simulink library "libControlTrimInputs"  (R2020b)
settings: Solver=VariableStepAuto  StartTime=0.0  StopTime=10.0  RelTol=1e-3
settings Model: Creator=caatay  LastModifiedBy=caatay

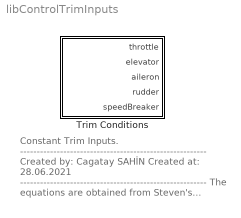
== system libControlTrimInputs ==
  note: Constant Trim Inputs.
      | --------------------------------------------------------
      | Created by: Cagatay SAHİN
      | Created at: 28.06.2021
      | --------------------------------------------------------
      | The equations are obtained from
      | Steven's textbook.
      | The reference book can be found in
      | "references folder".
      | --------------------------------------------------------
      | for question:
      | cagataysahin44@gmail.com
  Trim Conditions : Subsystem  mask(Flight Control System Model - Trim Input Library){throttle=outputs.trim.controls.throttle, elevator=outputs.trim.controls.elevator, aileron=outputs.trim.controls.aileron, rudder=outputs.trim.controls.rudder, sb=outputs.trim.controls.sb}
      mask prompts: throttle "Trimmed throttle value"; elevator "Trimmed elevator value"; aileron "Trimmed aileron value"; rudder "Trimmed rudder value"; sb "Trimmed sb value"
      mask help: Initialize trim input values for aircraft's steady-state flight
      mask Help:
      | This block is used for flight at steady-state trim inpıt.
      | --------------------------------------------------------------------------------------------------------------------------------------------------
      | Output of the function:
      | 	throttle: Trimmed throttle value.
      | 	elevator: Trimmed elevator value.
      | 	aileron: Trimmed aileron value.
      | 	rudder: Trimmed rudder value.
      | 	speedBreaker: Trimmed speedBreaker value.
      | --------------------------------------------------------------------------------------------------------------------------------------------------
      | All equations can be found in Steven's text book. Reference can be found in "literature" subfolder.
      | for question: "cagataysahin44@gmail.com"
      mask Display:
      | port_label('output',1,'\delta_{t}','texmode','on');
      | port_label('output',2,'\delta_{ele}','texmode','on');
      | port_label('output',3,'\delta_{ail}','texmode','on');
      | port_label('output',4,'\delta_{rud}','texmode','on');
      | port_label('output',5,'\delta_{sb}','texmode','on');

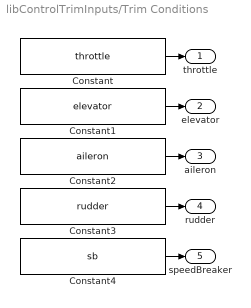
== system libControlTrimInputs/Trim Conditions ==
  Constant : Constant  Value=throttle
  Constant1 : Constant  Value=elevator
  Constant2 : Constant  Value=aileron
  Constant3 : Constant  Value=rudder
  Constant4 : Constant  Value=sb
  throttle : Outport  VectorParamsAs1DForOutWhenUnconnected=off
  elevator : Outport  Port=2  VectorParamsAs1DForOutWhenUnconnected=off
  aileron : Outport  Port=3  VectorParamsAs1DForOutWhenUnconnected=off
  rudder : Outport  Port=4  VectorParamsAs1DForOutWhenUnconnected=off
  speedBreaker : Outport  Port=5  VectorParamsAs1DForOutWhenUnconnected=off
  wires:
  Constant/1 -> throttle/1
  Constant3/1 -> rudder/1
  Constant2/1 -> aileron/1
  Constant1/1 -> elevator/1
  Constant4/1 -> speedBreaker/1
